simulink model "Verifica_LQR_05062026"  (R2025b)
settings: Solver=VariableStepAuto  StartTime=0.0  StopTime=50.0  RelTol=1e-3
undefined symbols (not defined in the file): A, B, D, K_LQR_i, K_LQR_x, r_lqr
settings Model: Creator=salvo  LastModifiedBy=salvo

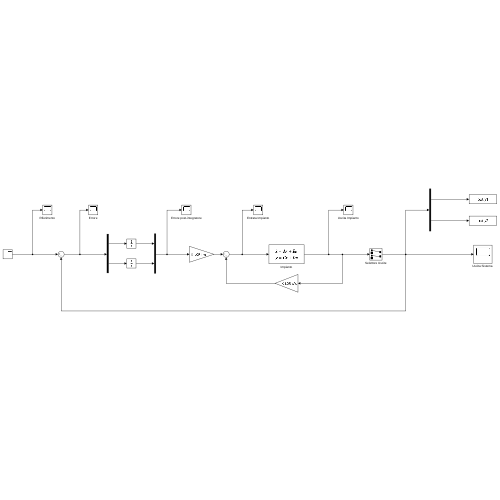
[thumbnail: Simulink's stored preview of the top-level diagram]
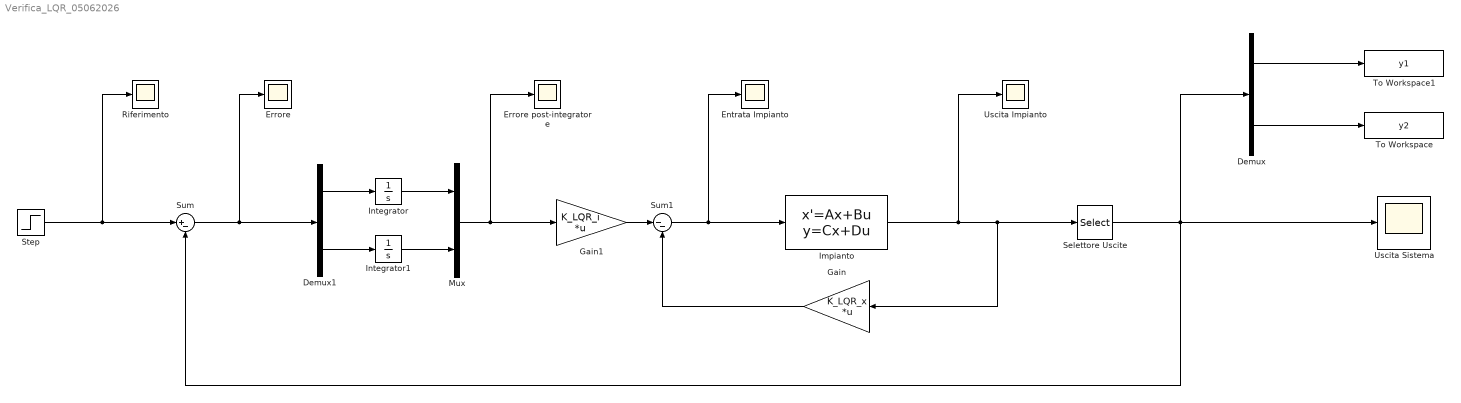
== system Verifica_LQR_05062026 ==
  Demux : Demux  Outputs=2
  Demux1 : Demux  Outputs=2
  Entrata Impianto : Scope
      settings: ActiveDisplayYMinimum=-1.4376526523532869  ActiveDisplayYMaximum=1.2030846532521546  DataLoggingVariableName=ScopeData5
  Errore : Scope
      settings: ActiveDisplayYMinimum=-0.29418197151740361  ActiveDisplayYMaximum=0.99885841903562977  DataLoggingVariableName=ScopeData3
  Errore post-integratore : Scope
      settings: ActiveDisplayYMinimum=0.033711477532444856  ActiveDisplayYMaximum=1.311208541216955  DataLoggingVariableName=ScopeData4
  Gain : Gain  Gain=K_LQR_x  Multiplication=Matrix(K*u)
  Gain1 : Gain  Gain=K_LQR_i  Multiplication=Matrix(K*u)
  Impianto : StateSpace  A=A  B=B  C=eye(4)  D=[D;zeros(2,2)]  InitialCondition=0
  Integrator : Integrator
  Integrator1 : Integrator
  Mux : Mux  Inputs=2
  Riferimento : Scope
      settings: ActiveDisplayYMinimum=-0.024457278627041362  ActiveDisplayYMaximum=0.27637012558434459  DataLoggingVariableName=ScopeData2
  Selettore Uscite : Selector  InputPortWidth=4  IndexOptions=Index vector (dialog)  Indices=[1 3]  OutputSizes=1
  Step : Step  After=r_lqr  SampleTime=0  VectorParams1D=off
  Sum : Sum  Inputs=|+-
  Sum1 : Sum  Inputs=|--
  To Workspace : ToWorkspace  VariableName=y2  SaveFormat=Timeseries  SampleTime=-1
  To Workspace1 : ToWorkspace  VariableName=y1  SaveFormat=Timeseries  SampleTime=-1
  Uscita Impianto : Scope
      settings: ActiveDisplayYMinimum=-18.453614759389517  ActiveDisplayYMaximum=16.838996566087474
  "Uscita Sistema " : Scope
      settings: ActiveDisplayYMinimum=-0.30257780139312912  ActiveDisplayYMaximum=0.53519599442223553
  wires:
  Gain1/1 -> Sum1/1
  Gain/1 -> Sum1/2
  Impianto/1 -> Gain/1, Selettore Uscite/1, Uscita Impianto/1
  Sum1/1 -> Impianto/1, Entrata Impianto/1
  Integrator/1 -> Mux/1
  Integrator1/1 -> Mux/2
  Mux/1 -> Gain1/1, Errore post-integratore/1
  Demux1/2 -> Integrator1/1
  Demux1/1 -> Integrator/1
  Step/1 -> Riferimento/1, Sum/1
  Sum/1 -> Errore/1, Demux1/1
  Selettore Uscite/1 -> "Uscita Sistema "/1, Demux/1, Sum/2
  Demux/2 -> To Workspace/1
  Demux/1 -> To Workspace1/1
